simulink model "Model_pf_regulacije"  (R2024a)
settings: Solver=VariableStepAuto  StartTime=0.0  StopTime=Tsim  RelTol=1e-3
values from neighbouring files (symbols this model uses):
  Cv = [c1 c0]    [Model_pf_regulacije_eng.m]
  Fn = 50    [Model_pf_regulacije_eng.m]
  Lv = [l1 l0]    [Model_pf_regulacije_eng.m]
  n_LG2_CHM = 13    [Model_pf_regulacije_eng.m]
  n_LG2_LG3 = 2    [Model_pf_regulacije_eng.m]
  n_LG3_CHM = 6    [Model_pf_regulacije_eng.m]
  n_LG3_LG4 = 2    [Model_pf_regulacije_eng.m]
  n_LG4_CHM = 8    [Model_pf_regulacije_eng.m]
  P_LG31loc = 5e6    (= 5000000)    [Model_pf_regulacije_eng.m]
  PSStype = 1    [Model_pf_regulacije_eng.m]
  Rv = [r1 r0]    [Model_pf_regulacije_eng.m]
  t_ispad_LG31 = 100    [Model_pf_regulacije_eng.m]
  t_ispad_voda_LG2_LG3 = 1e6    (= 1000000)    [Model_pf_regulacije_eng.m]
  t_povecanje_potrosnje = 1e6    (= 1000000)    [Model_pf_regulacije_eng.m]
  Ts = 50e-6    (= 5e-05)    [Model_pf_regulacije_eng.m]
  Vg = 13.8e3    (= 13800)    [Model_pf_regulacije_eng.m]
  Vrms = 230e3    (= 230000)    [Model_pf_regulacije_eng.m]
undefined symbols (not defined in the file or in its folder): D1, Delta
libraries: spsThreePhaseParallelRLCLoadLib x6, spsDistributedParametersLineLib x5, spsThreePhaseTransformerTwoWindingsLib x4, spsSynchronousMachinepuStandardLib x4, spsRMSLib x4, spsExcitationSystemLib x4, spsHydraulicTurbineandGovernorLib x4, spsGenericPowerSystemStabilizerLib x4, spsMultiBandPowerSystemStabilizerLib x4, spsThreePhaseBreakerLib x3, spsThreePhaseSeriesRLCLoadLib x2, dspstat3 x2
(part 2 of 2)

== system Model_pf_regulacije/Regulators3/Turbine  & Excitation Regulators Mac2/Stabilizer ==
  Pm : Inport
  Pe : Inport  Port=2
  dw : Inport  Port=3
  Generic Power System Stabilizer : spsGenericPowerSystemStabilizerLib/Generic Power System Stabilizer  Tsensor=15e-3  K=2.5  Twashout=1  Tleadlag1="[0.06  1]"  Tleadlag2="[0  0]"  VSlimits=[-0.15 0.15]  Vinit=0  Plot_On=off  MagdB_On=on  FreqRange=logspace(-2,2,500)
  Ground1 : Ground
  Multi-Band Power System Stabilizer : spsMultiBandPowerSystemStabilizerLib/Multi-Band Power System Stabilizer  OperationMode=Simplified settings  Kg=0.7  GL=[0.2 10]  GI=[0.9 30]  GH=[12.0 115]  GLd=[66 66 9.4]  TcLF=[1.667 2 0 0 0 0 2 2.4 0 0 0 0 1 1]  GId=[66 66 47.6]  TcIF=[1 1 0.25 0.3 0 0 1 1 0.3 0.36 0 0 0 0]  GHd=[66 66 233]  TcHF="[0.01 0.012 0 0 0 0  0.012 0.0144 0 0 0 0 1 1]"  LIM=[.075 .15 .15 .15]  Plot_On=off  MagdB_On=on  FreqRange=logspace(-2,2,500)
  Multiport Switch : MultiPortSwitch
  PSS1 : Constant  Value=PSStype
  Sum2 : Sum  Inputs=+-  InputSameDT=on  SaturateOnIntegerOverflow=on  OutDataTypeStr=Inherit: Same as first input
  Stab : Outport  InitialOutput=0  VectorParamsAs1DForOutWhenUnconnected=off
  wires:
  Multi-Band Power System Stabilizer/1 -> Multiport Switch/4
  dw/1 -> Multi-Band Power System Stabilizer/1
  PSS1/1 -> Multiport Switch/1
  Ground1/1 -> Multiport Switch/2
  Pe/1 -> Sum2/2
  Pm/1 -> Sum2/1
  Sum2/1 -> Generic Power System Stabilizer/1
  Generic Power System Stabilizer/1 -> Multiport Switch/3
  Multiport Switch/1 -> Stab/1

== system Model_pf_regulacije/Regulators4/Turbine  & Excitation Regulators Mac2/Stabilizer ==
  Pm : Inport
  Pe : Inport  Port=2
  dw : Inport  Port=3
  Generic Power System Stabilizer : spsGenericPowerSystemStabilizerLib/Generic Power System Stabilizer  Tsensor=15e-3  K=2.5  Twashout=1  Tleadlag1="[0.06  1]"  Tleadlag2="[0  0]"  VSlimits=[-0.15 0.15]  Vinit=0  Plot_On=off  MagdB_On=on  FreqRange=logspace(-2,2,500)
  Ground1 : Ground
  Multi-Band Power System Stabilizer : spsMultiBandPowerSystemStabilizerLib/Multi-Band Power System Stabilizer  OperationMode=Simplified settings  Kg=0.7  GL=[0.2 10]  GI=[0.9 30]  GH=[12.0 115]  GLd=[66 66 9.4]  TcLF=[1.667 2 0 0 0 0 2 2.4 0 0 0 0 1 1]  GId=[66 66 47.6]  TcIF=[1 1 0.25 0.3 0 0 1 1 0.3 0.36 0 0 0 0]  GHd=[66 66 233]  TcHF="[0.01 0.012 0 0 0 0  0.012 0.0144 0 0 0 0 1 1]"  LIM=[.075 .15 .15 .15]  Plot_On=off  MagdB_On=on  FreqRange=logspace(-2,2,500)
  Multiport Switch : MultiPortSwitch
  PSS1 : Constant  Value=PSStype
  Sum2 : Sum  Inputs=+-  InputSameDT=on  SaturateOnIntegerOverflow=on  OutDataTypeStr=Inherit: Same as first input
  Stab : Outport  InitialOutput=0  VectorParamsAs1DForOutWhenUnconnected=off
  wires:
  Multi-Band Power System Stabilizer/1 -> Multiport Switch/4
  Multiport Switch/1 -> Stab/1
  Generic Power System Stabilizer/1 -> Multiport Switch/3
  Sum2/1 -> Generic Power System Stabilizer/1
  Pm/1 -> Sum2/1
  Pe/1 -> Sum2/2
  Ground1/1 -> Multiport Switch/2
  PSS1/1 -> Multiport Switch/1
  dw/1 -> Multi-Band Power System Stabilizer/1
